simulink library "PC_Simulator_Lib"  (Simulink 8.2)
settings: Solver=ode45  StartTime=0.0  StopTime=10.0  RelTol=1e-3
values from neighbouring files (symbols this model uses):
  data = [r1 r2 r3 r4 L1 L2 L3 L4]    [strasse_Bedatung_HNI_ITI.m]
  distSameLane = 60    [InitialisationsEnv.m]
  eng_speed = [0 60 120 180 240 300 360 420 480 540 600 660 ... (101 elements, 1x101)]    [engine_table.mat]    (also in motor_parameter_calc.m = omega)
  Heading_init = 0    [Start.m]
  inertiaLateral = 25*(radiusWheel)^2    (= 4.129024)    [Start.m]
  laneWidth = 3.6    [InitialisationsEnv.m]    (also in strasse_Bedatung_HNI_ITI.m)
  omega_engine = [0.000000 150.000000 500.000000 1000.000000 1500.000000 2000.000000 2500.000000 3000.000000 3500.000000 4000.000000 4500.000000 5000.000000 5500.000000 6000.000000]    [friction_tables.m]
  omega_max = 6000    [engine_table.mat]    (also in motor_parameter_calc.m)
  omega_wheel = [0 20 40 60 80 100 122 143.7 164]    [friction_tables.m]
  para_Fellow_8_Points = ADAS.Fellow_8_Points    [ADAS_parameters.m]
  position_start_x = [x1 x2 x3 x4 x5 x6 x7]    [strasse_Bedatung_HNI_ITI.m]
  position_start_y = [y1 y2 y3 y4 y5 y6 y7]    [strasse_Bedatung_HNI_ITI.m]
  rad3rdLine = 57.2    [InitialisationsEnv.m]    (also in strasse_Bedatung_HNI_ITI.m)
  radiusWheel = 16*2.54/100    (= 0.4064)    [Start.m]
  s_values = [S1 S2 S3 S4 S5 S6 S7]    [strasse_Bedatung_HNI_ITI.m]
  segmentLimits = [segment1EndThirdLine                   segment2EndThirdLine                   segment3EndThirdLine                   segment4EndThirdLine                   segment5EndThirdLine                   segment6EndThirdLine                   segment7EndThirdLine                   segment8EndThirdLine                   ]    [InitialisationsEnv.m]    (also in strasse_Bedatung_HNI_ITI.m)
  setPosT = [-1.8 -5.4 -1.8 -5.4 -1.8 -5.4 -1.8 -5.4 -1.8 -5.4]    [InitialisationsEnv.m]
  torque = [297.089227105 300.997600937 304.800343044 308.497453426 312.088932082 315.574779014 318.95499422 322.229577701 325.398529457 328.461849487 331.419537793 334.271594373 ... (101 elements, 1x101)]    [engine_table.mat]    (also in motor_parameter_calc.m = g)
  Torque_lost = [0.000000 -8.777780 -15.000000 -26.800000 -29.600000 -32.700000 -35.900000 -39.300000 -42.800000 -46.500000 -50.300000 -54.300000 -58.500000 -62.800000 ]*0.6    [friction_tables.m]
  Torque_lost_wheel = [0.8 0.8 0.75 0.7 0.4 0.3 0.2 0.07 0.07]*0.2    [friction_tables.m]
  X_init = 0    [Start.m]
  Y_init = 1.8    [Start.m]
  Z_init = 0    [Start.m]
undefined symbols (not defined in the file or in its folder): Acc_Pedal, ADAS, Brake_Pedal, Joystick, Newton, Para, Raphson, Standard_Devices, Steering_Wheel_Angle, UDP_Protocol
libraries: simulink x43, rtwinlib x7, dspnetwork x2, simulink_extras x1, vrlib x1
(part 6 of 13)

== system PC_Simulator_Lib/Comunication_with_visualisation_Realtime/Subsystem2/Subsystem17 ==
  v[m|s] : Inport
  Gain : Gain  Gain=1/radiusWheel
  Integrator : Integrator
  Wheels_Rotation_Angle[rad] : Outport
  wires:
  Integrator/1 -> Wheels_Rotation_Angle[rad]/1
  v[m|s]/1 -> Gain/1
  Gain/1 -> Integrator/1

== system PC_Simulator_Lib/Comunication_with_visualisation_Realtime/Subsystem2/Subsystem18 ==
  v[m|s] : Inport
  Gain : Gain  Gain=1/radiusWheel
  Integrator : Integrator
  Wheels_Rotation_Angle[rad] : Outport
  wires:
  Gain/1 -> Integrator/1
  v[m|s]/1 -> Gain/1
  Integrator/1 -> Wheels_Rotation_Angle[rad]/1

== system PC_Simulator_Lib/Comunication_with_visualisation_Realtime/Subsystem2/Subsystem19 ==
  v[m|s] : Inport
  Gain : Gain  Gain=1/radiusWheel
  Integrator : Integrator
  Wheels_Rotation_Angle[rad] : Outport
  wires:
  Integrator/1 -> Wheels_Rotation_Angle[rad]/1
  v[m|s]/1 -> Gain/1
  Gain/1 -> Integrator/1

== system PC_Simulator_Lib/Comunication_with_visualisation_Realtime/Subsystem2/Subsystem2 ==
  In1 : Inport
  Constant9 : Constant  Value=Z_init
  Sum : Sum  Inputs=|++
  Out1 : Outport
  wires:
  In1/1 -> Sum/1
  Constant9/1 -> Sum/2
  Sum/1 -> Out1/1

== system PC_Simulator_Lib/Comunication_with_visualisation_Realtime/Subsystem2/Subsystem20 ==
  v[m|s] : Inport
  Gain : Gain  Gain=1/radiusWheel
  Integrator : Integrator
  Wheels_Rotation_Angle[rad] : Outport
  wires:
  Gain/1 -> Integrator/1
  v[m|s]/1 -> Gain/1
  Integrator/1 -> Wheels_Rotation_Angle[rad]/1

== system PC_Simulator_Lib/Comunication_with_visualisation_Realtime/Subsystem2/Subsystem3 ==
  FeedBack : Inport
  Mux : Mux  Inputs=14
  Terminator : Terminator
  zeros{7..10} (4 alike) : Constant  Value=0
  zeros12 : Constant
  Enablble_Fellow_Vehicles[bool] : Outport
  wires:
  Mux/1 -> Enablble_Fellow_Vehicles[bool]/1
  zeros12/1 -> Mux/2, Mux/6, Mux/7, Mux/8, Mux/9, Mux/10, Mux/5, Mux/4, Mux/3, Mux/1
  zeros7/1 -> Mux/12
  zeros8/1 -> Mux/11
  zeros9/1 -> Mux/14
  zeros10/1 -> Mux/13
  FeedBack/1 -> Terminator/1

== system PC_Simulator_Lib/Comunication_with_visualisation_Realtime/Subsystem2/Subsystem4 ==
  In1 : Inport
  Constant9 : Constant  Value=Z_init
  Sum : Sum  Inputs=|++
  Out1 : Outport
  wires:
  Sum/1 -> Out1/1
  Constant9/1 -> Sum/2
  In1/1 -> Sum/1

== system PC_Simulator_Lib/Comunication_with_visualisation_Realtime/Subsystem2/Subsystem5 ==
  In1 : Inport
  Constant9 : Constant  Value=Z_init
  Sum : Sum  Inputs=|++
  Out1 : Outport
  wires:
  In1/1 -> Sum/1
  Constant9/1 -> Sum/2
  Sum/1 -> Out1/1

== system PC_Simulator_Lib/Comunication_with_visualisation_Realtime/Subsystem2/Subsystem6 ==
  In1 : Inport
  Constant9 : Constant  Value=Z_init
  Sum : Sum  Inputs=|++
  Out1 : Outport
  wires:
  Sum/1 -> Out1/1
  Constant9/1 -> Sum/2
  In1/1 -> Sum/1

== system PC_Simulator_Lib/Comunication_with_visualisation_Realtime/Subsystem2/Subsystem7 ==
  In1 : Inport
  Constant9 : Constant  Value=Z_init
  Sum : Sum  Inputs=|++
  Out1 : Outport
  wires:
  In1/1 -> Sum/1
  Constant9/1 -> Sum/2
  Sum/1 -> Out1/1

== system PC_Simulator_Lib/Comunication_with_visualisation_Realtime/Subsystem2/Subsystem8 ==
  In1 : Inport
  Constant9 : Constant  Value=Z_init
  Sum : Sum  Inputs=|++
  Out1 : Outport
  wires:
  Sum/1 -> Out1/1
  Constant9/1 -> Sum/2
  In1/1 -> Sum/1

== system PC_Simulator_Lib/Comunication_with_visualisation_Realtime/Subsystem2/Subsystem9 ==
  In1 : Inport
  Constant9 : Constant  Value=Z_init
  Sum : Sum  Inputs=|++
  Out1 : Outport
  wires:
  In1/1 -> Sum/1
  Constant9/1 -> Sum/2
  Sum/1 -> Out1/1

== system PC_Simulator_Lib/Comunication_with_visualisation_Realtime_new_version/Maping_Block/Subsystem ==
  Vehicle_1_Vector : Inport
  Vehicle_2_Vector : Inport  Port=2
  Vehicle_3_Vector : Inport  Port=3
  Vehicle_4_Vector : Inport  Port=4
  Vehicle_5_Vector : Inport  Port=5
  Vehicle_6_Vector : Inport  Port=6
  Vehicle_7_Vector : Inport  Port=7
  Vehicle_8_Vector : Inport  Port=8
  Vehicle_9_Vector : Inport  Port=9
  Vehicle_10_Vector : Inport  Port=10
  Vehicle_11_Vector : Inport  Port=11
  Vehicle_12_Vector : Inport  Port=12
  Vehicle_13_Vector : Inport  Port=13
  Vehicle_14_Vector : Inport  Port=14
  Bus Creator : BusCreator  Inputs=14
  Bus Selector : BusSelector  OutputSignals=Vehicle_1_Vector.Vehicle_1_x[m],Vehicle_2_Vector.Vehicle_2_x[m],Vehicle_3_Vector.Vehicle_3_x[m],Vehicle_4_Vector3.Vehicle_4_x[m],Vehicle_5_Vector.Vehicle_5_x[m],Vehicle_6_Vector.Vehicle_6_x[m],Vehicle_7_Vector.Vehicle_7_x[m],Vehicle_8_Vector.Vehicle_8_x[m],Vehicle_9_Vector.Vehicle_9_x[m],Vehicle_10_Vector.Vehicle_10_x[m],Vehicle_11_Vector.Vehicle_11_x[m],Vehicle_12_Vector.Vehicle_12_x[m],Vehicle_13_Vector.Vehicle_13_x[m],Vehicle_14_Vector.Vehicle_14_x[m]
  Bus Selector1 : BusSelector  OutputSignals=Vehicle_1_Vector.Vehicle_1_y[m],Vehicle_2_Vector.Vehicle_2_y[m],Vehicle_3_Vector.Vehicle_3_y[m],Vehicle_4_Vector3.Vehicle_4_y[m],Vehicle_5_Vector.Vehicle_5_y[m],Vehicle_6_Vector.Vehicle_6_y[m],Vehicle_7_Vector.Vehicle_7_y[m],Vehicle_8_Vector.Vehicle_8_y[m],Vehicle_9_Vector.Vehicle_9_y[m],Vehicle_10_Vector.Vehicle_10_y[m],Vehicle_11_Vector.Vehicle_11_y[m],Vehicle_12_Vector.Vehicle_12_y[m],Vehicle_13_Vector.Vehicle_13_y[m],Vehicle_14_Vector.Vehicle_14_y[m]
  Bus Selector2 : BusSelector  OutputSignals=Vehicle_1_Vector.Vehicle_1_z[m],Vehicle_2_Vector.Vehicle_2_z[m],Vehicle_3_Vector.Vehicle_3_z[m],Vehicle_4_Vector3.Vehicle_4_z[m],Vehicle_5_Vector.Vehicle_5_z[m],Vehicle_6_Vector.Vehicle_6_z[m],Vehicle_7_Vector.Vehicle_7_z[m],Vehicle_8_Vector.Vehicle_8_z[m],Vehicle_9_Vector.Vehicle_9_z[m],Vehicle_10_Vector.Vehicle_10_z[m],Vehicle_11_Vector.Vehicle_11_z[m],Vehicle_12_Vector.Vehicle_12_z[m],Vehicle_13_Vector.Vehicle_13_z[m],Vehicle_14_Vector.Vehicle_14_z[m]
  Bus Selector3 : BusSelector  OutputSignals=Vehicle_1_Vector.Vehicle_1_Gear_Angle[deg],Vehicle_2_Vector.Vehicle_2_Gear_Angle[deg],Vehicle_3_Vector.Vehicle_3_Gear_Angle[deg],Vehicle_4_Vector3.Vehicle_4_Gear_Angle[deg],Vehicle_5_Vector.Vehicle_5_Gear_Angle[deg],Vehicle_6_Vector.Vehicle_6_Gear_Angle[deg],Vehicle_7_Vector.Vehicle_7_Gear_Angle[deg],Vehicle_8_Vector.Vehicle_8_Gear_Angle[deg],Vehicle_9_Vector.Vehicle_9_Gear_Angle[deg],Vehicle_10_Vector.Vehicle_10_Gear_Angle[deg],Vehicle_11_Vector.Vehicle_11_Gear_Angle[deg],Vehicle_12_Vector.Vehicle_12_Gear_Angle[deg],Vehicle_13_Vector.Vehicle_13_Gear_Angle[deg],Vehicle_14_Vector.Vehicle_14_Gear_Angle[deg]
  Bus Selector4 : BusSelector  OutputSignals=Vehicle_1_Vector.Vehicle_1_Wheels_Rotation_Angle[deg],Vehicle_2_Vector.Vehicle_2_Wheels_Rotation_Angle[deg],Vehicle_3_Vector.Vehicle_3_Wheels_Rotation_Angle[deg],Vehicle_4_Vector3.Vehicle_4_Wheels_Rotation_Angle[deg],Vehicle_5_Vector.Vehicle_5_Wheels_Rotation_Angle[deg],Vehicle_6_Vector.Vehicle_6_Wheels_Rotation_Angle[deg],Vehicle_7_Vector.Vehicle_7_Wheels_Rotation_Angle[deg],Vehicle_8_Vector.Vehicle_8_Wheels_Rotation_Angle[deg],Vehicle_9_Vector.Vehicle_9_Wheels_Rotation_Angle[deg],Vehicle_10_Vector.Vehicle_10_Wheels_Rotation_Angle[deg],Vehicle_11_Vector.Vehicle_11_Wheels_Rotation_Angle[deg],Vehicle_12_Vector.Vehicle_12_Wheels_Rotation_Angle[deg],Vehicle_13_Vector.Vehicle_13_Wheels_Rotation_Angle[deg],Vehicle_14_Vector.Vehicle_14_Wheels_Rotation_Angle[deg]
  Mux{,1..4} (5 alike) : Mux  Inputs=14
  Fellow_Vehicles_x_Vector_14[m] : Outport
  Fellow_Vehicles_y_Vector_14[m] : Outport  Port=2
  Fellow_Vehicles_z_Vector_14[m] : Outport  Port=3
  Fellow_Vehicles_Gear_Angle_Vector_14[deg] : Outport  Port=4
  Fellow_Vehicles_Wheel_Angle_Vector_14[deg] : Outport  Port=5
  wires:
  Mux4/1 -> Fellow_Vehicles_Wheel_Angle_Vector_14[deg]/1
  Mux3/1 -> Fellow_Vehicles_Gear_Angle_Vector_14[deg]/1
  Mux2/1 -> Fellow_Vehicles_z_Vector_14[m]/1
  Mux1/1 -> Fellow_Vehicles_y_Vector_14[m]/1
  Mux/1 -> Fellow_Vehicles_x_Vector_14[m]/1
  Bus Selector4/1 -> Mux4/1  "<Vehicle_1_Wheels_Rotation_Angle[deg]>"
  Bus Selector4/2 -> Mux4/2  "<Vehicle_2_Wheels_Rotation_Angle[deg]>"
  Bus Selector4/14 -> Mux4/14  "<Vehicle_14_Wheels_Rotation_Angle[deg]>"
  Bus Selector4/3 -> Mux4/3  "<Vehicle_3_Wheels_Rotation_Angle[deg]>"
  Bus Selector4/13 -> Mux4/13  "<Vehicle_13_Wheels_Rotation_Angle[deg]>"
  Bus Selector4/4 -> Mux4/4  "<Vehicle_4_Wheels_Rotation_Angle[deg]>"
  Bus Selector4/12 -> Mux4/12  "<Vehicle_12_Wheels_Rotation_Angle[deg]>"
  Bus Selector4/5 -> Mux4/5  "<Vehicle_5_Wheels_Rotation_Angle[deg]>"
  Bus Selector4/11 -> Mux4/11  "<Vehicle_11_Wheels_Rotation_Angle[deg]>"
  Bus Selector4/6 -> Mux4/6  "<Vehicle_6_Wheels_Rotation_Angle[deg]>"
  Bus Selector4/10 -> Mux4/10  "<Vehicle_10_Wheels_Rotation_Angle[deg]>"
  Bus Selector4/7 -> Mux4/7  "<Vehicle_7_Wheels_Rotation_Angle[deg]>"
  Bus Selector4/9 -> Mux4/9  "<Vehicle_9_Wheels_Rotation_Angle[deg]>"
  Bus Selector4/8 -> Mux4/8  "<Vehicle_8_Wheels_Rotation_Angle[deg]>"
  Bus Creator/1 -> Bus Selector/1, Bus Selector1/1, Bus Selector2/1, Bus Selector3/1, Bus Selector4/1
  Bus Selector3/1 -> Mux3/1  "<Vehicle_1_Gear_Angle[deg]>"
  Bus Selector3/2 -> Mux3/2  "<Vehicle_2_Gear_Angle[deg]>"
  Bus Selector3/14 -> Mux3/14  "<Vehicle_14_Gear_Angle[deg]>"
  Bus Selector3/3 -> Mux3/3  "<Vehicle_3_Gear_Angle[deg]>"
  Bus Selector3/13 -> Mux3/13  "<Vehicle_13_Gear_Angle[deg]>"
  Bus Selector3/4 -> Mux3/4  "<Vehicle_4_Gear_Angle[deg]>"
  Bus Selector3/12 -> Mux3/12  "<Vehicle_12_Gear_Angle[deg]>"
  Bus Selector3/5 -> Mux3/5  "<Vehicle_5_Gear_Angle[deg]>"
  Bus Selector3/11 -> Mux3/11  "<Vehicle_11_Gear_Angle[deg]>"
  Bus Selector3/6 -> Mux3/6  "<Vehicle_6_Gear_Angle[deg]>"
  Bus Selector3/10 -> Mux3/10  "<Vehicle_10_Gear_Angle[deg]>"
  Bus Selector3/7 -> Mux3/7  "<Vehicle_7_Gear_Angle[deg]>"
  Bus Selector3/9 -> Mux3/9  "<Vehicle_9_Gear_Angle[deg]>"
  Bus Selector3/8 -> Mux3/8  "<Vehicle_8_Gear_Angle[deg]>"
  Bus Selector2/1 -> Mux2/1  "<Vehicle_1_z[m]>"
  Bus Selector2/2 -> Mux2/2  "<Vehicle_2_z[m]>"
  Bus Selector2/14 -> Mux2/14  "<Vehicle_14_z[m]>"
  Bus Selector2/3 -> Mux2/3  "<Vehicle_3_z[m]>"
  Bus Selector2/13 -> Mux2/13  "<Vehicle_13_z[m]>"
  Bus Selector2/4 -> Mux2/4  "<Vehicle_4_z[m]>"
  Bus Selector2/12 -> Mux2/12  "<Vehicle_12_z[m]>"
  Bus Selector2/5 -> Mux2/5  "<Vehicle_5_z[m]>"
  Bus Selector2/11 -> Mux2/11  "<Vehicle_11_z[m]>"
  Bus Selector2/6 -> Mux2/6  "<Vehicle_6_z[m]>"
  Bus Selector2/10 -> Mux2/10  "<Vehicle_10_z[m]>"
  Bus Selector2/7 -> Mux2/7  "<Vehicle_7_z[m]>"
  Bus Selector2/9 -> Mux2/9  "<Vehicle_9_z[m]>"
  Bus Selector2/8 -> Mux2/8  "<Vehicle_8_z[m]>"
  Bus Selector1/1 -> Mux1/1  "<Vehicle_1_y[m]>"
  Bus Selector1/2 -> Mux1/2  "<Vehicle_2_y[m]>"
  Bus Selector1/14 -> Mux1/14  "<Vehicle_14_y[m]>"
  Bus Selector1/3 -> Mux1/3  "<Vehicle_3_y[m]>"
  Bus Selector1/13 -> Mux1/13  "<Vehicle_13_y[m]>"
  Bus Selector1/4 -> Mux1/4  "<Vehicle_4_y[m]>"
  Bus Selector1/12 -> Mux1/12  "<Vehicle_12_y[m]>"
  Bus Selector1/5 -> Mux1/5  "<Vehicle_5_y[m]>"
  Bus Selector1/11 -> Mux1/11  "<Vehicle_11_y[m]>"
  Bus Selector1/6 -> Mux1/6  "<Vehicle_6_y[m]>"
  Bus Selector1/10 -> Mux1/10  "<Vehicle_10_y[m]>"
  Bus Selector1/7 -> Mux1/7  "<Vehicle_7_y[m]>"
  Bus Selector1/9 -> Mux1/9  "<Vehicle_9_y[m]>"
  Bus Selector1/8 -> Mux1/8  "<Vehicle_8_y[m]>"
  Bus Selector/1 -> Mux/1  "<Vehicle_1_x[m]>"
  Bus Selector/2 -> Mux/2  "<Vehicle_2_x[m]>"
  Bus Selector/14 -> Mux/14  "<Vehicle_14_x[m]>"
  Bus Selector/3 -> Mux/3  "<Vehicle_3_x[m]>"
  Bus Selector/13 -> Mux/13  "<Vehicle_13_x[m]>"
  Bus Selector/4 -> Mux/4  "<Vehicle_4_x[m]>"
  Bus Selector/12 -> Mux/12  "<Vehicle_12_x[m]>"
  Bus Selector/5 -> Mux/5  "<Vehicle_5_x[m]>"
  Bus Selector/11 -> Mux/11  "<Vehicle_11_x[m]>"
  Bus Selector/6 -> Mux/6  "<Vehicle_6_x[m]>"
  Bus Selector/10 -> Mux/10  "<Vehicle_10_x[m]>"
  Bus Selector/7 -> Mux/7  "<Vehicle_7_x[m]>"
  Bus Selector/9 -> Mux/9  "<Vehicle_9_x[m]>"
  Bus Selector/8 -> Mux/8  "<Vehicle_8_x[m]>"
  Vehicle_14_Vector/1 -> Bus Creator/14
  Vehicle_12_Vector/1 -> Bus Creator/12
  Vehicle_11_Vector/1 -> Bus Creator/11
  Vehicle_9_Vector/1 -> Bus Creator/9
  Vehicle_10_Vector/1 -> Bus Creator/10
  Vehicle_13_Vector/1 -> Bus Creator/13
  Vehicle_8_Vector/1 -> Bus Creator/8
  Vehicle_7_Vector/1 -> Bus Creator/7
  Vehicle_6_Vector/1 -> Bus Creator/6
  Vehicle_5_Vector/1 -> Bus Creator/5
  Vehicle_4_Vector/1 -> Bus Creator/4
  Vehicle_3_Vector/1 -> Bus Creator/3
  Vehicle_2_Vector/1 -> Bus Creator/2
  Vehicle_1_Vector/1 -> Bus Creator/1

== system PC_Simulator_Lib/Comunication_with_visualisation_Realtime_new_version/Subsystem2/Subsystem ==
  In1 : Inport
  Constant9 : Constant  Value=0.8
  Sum : Sum  Inputs=|++
  Out1 : Outport
  wires:
  Sum/1 -> Out1/1
  Constant9/1 -> Sum/2
  In1/1 -> Sum/1

== system PC_Simulator_Lib/Comunication_with_visualisation_Realtime_new_version/Subsystem2/Subsystem1 ==
  In1 : Inport
  Constant9 : Constant  Value=Z_init
  Sum : Sum  Inputs=|++
  Out1 : Outport
  wires:
  In1/1 -> Sum/1
  Constant9/1 -> Sum/2
  Sum/1 -> Out1/1

== system PC_Simulator_Lib/Comunication_with_visualisation_Realtime_new_version/Subsystem2/Subsystem10 ==
  In1 : Inport
  Constant9 : Constant  Value=Z_init
  Sum : Sum  Inputs=|++
  Out1 : Outport
  wires:
  In1/1 -> Sum/1
  Constant9/1 -> Sum/2
  Sum/1 -> Out1/1

== system PC_Simulator_Lib/Comunication_with_visualisation_Realtime_new_version/Subsystem2/Subsystem11 ==
  v[m|s] : Inport
  Gain : Gain  Gain=1/radiusWheel
  Integrator : Integrator
  Wheels_Rotation_Angle[rad] : Outport
  wires:
  Gain/1 -> Integrator/1
  v[m|s]/1 -> Gain/1
  Integrator/1 -> Wheels_Rotation_Angle[rad]/1

== system PC_Simulator_Lib/Comunication_with_visualisation_Realtime_new_version/Subsystem2/Subsystem12 ==
  v[m|s] : Inport
  Gain : Gain  Gain=1/radiusWheel
  Integrator : Integrator
  Wheels_Rotation_Angle[rad] : Outport
  wires:
  Integrator/1 -> Wheels_Rotation_Angle[rad]/1
  v[m|s]/1 -> Gain/1
  Gain/1 -> Integrator/1

== system PC_Simulator_Lib/Comunication_with_visualisation_Realtime_new_version/Subsystem2/Subsystem13 ==
  v[m|s] : Inport
  Gain : Gain  Gain=1/radiusWheel
  Integrator : Integrator
  Wheels_Rotation_Angle[rad] : Outport
  wires:
  Gain/1 -> Integrator/1
  v[m|s]/1 -> Gain/1
  Integrator/1 -> Wheels_Rotation_Angle[rad]/1

== system PC_Simulator_Lib/Comunication_with_visualisation_Realtime_new_version/Subsystem2/Subsystem14 ==
  v[m|s] : Inport
  Gain : Gain  Gain=1/radiusWheel
  Integrator : Integrator
  Wheels_Rotation_Angle[rad] : Outport
  wires:
  Integrator/1 -> Wheels_Rotation_Angle[rad]/1
  v[m|s]/1 -> Gain/1
  Gain/1 -> Integrator/1

== system PC_Simulator_Lib/Comunication_with_visualisation_Realtime_new_version/Subsystem2/Subsystem15 ==
  v[m|s] : Inport
  Gain : Gain  Gain=1/radiusWheel
  Integrator : Integrator
  Wheels_Rotation_Angle[rad] : Outport
  wires:
  Gain/1 -> Integrator/1
  v[m|s]/1 -> Gain/1
  Integrator/1 -> Wheels_Rotation_Angle[rad]/1

== system PC_Simulator_Lib/Comunication_with_visualisation_Realtime_new_version/Subsystem2/Subsystem16 ==
  v[m|s] : Inport
  Gain : Gain  Gain=1/radiusWheel
  Integrator : Integrator
  Wheels_Rotation_Angle[rad] : Outport
  wires:
  Integrator/1 -> Wheels_Rotation_Angle[rad]/1
  v[m|s]/1 -> Gain/1
  Gain/1 -> Integrator/1

== system PC_Simulator_Lib/Comunication_with_visualisation_Realtime_new_version/Subsystem2/Subsystem17 ==
  v[m|s] : Inport
  Gain : Gain  Gain=1/radiusWheel
  Integrator : Integrator
  Wheels_Rotation_Angle[rad] : Outport
  wires:
  Gain/1 -> Integrator/1
  v[m|s]/1 -> Gain/1
  Integrator/1 -> Wheels_Rotation_Angle[rad]/1

== system PC_Simulator_Lib/Comunication_with_visualisation_Realtime_new_version/Subsystem2/Subsystem18 ==
  v[m|s] : Inport
  Gain : Gain  Gain=1/radiusWheel
  Integrator : Integrator
  Wheels_Rotation_Angle[rad] : Outport
  wires:
  Integrator/1 -> Wheels_Rotation_Angle[rad]/1
  v[m|s]/1 -> Gain/1
  Gain/1 -> Integrator/1

== system PC_Simulator_Lib/Comunication_with_visualisation_Realtime_new_version/Subsystem2/Subsystem19 ==
  v[m|s] : Inport
  Gain : Gain  Gain=1/radiusWheel
  Integrator : Integrator
  Wheels_Rotation_Angle[rad] : Outport
  wires:
  Gain/1 -> Integrator/1
  v[m|s]/1 -> Gain/1
  Integrator/1 -> Wheels_Rotation_Angle[rad]/1

== system PC_Simulator_Lib/Comunication_with_visualisation_Realtime_new_version/Subsystem2/Subsystem2 ==
  In1 : Inport
  Constant9 : Constant  Value=Z_init
  Sum : Sum  Inputs=|++
  Out1 : Outport
  wires:
  Sum/1 -> Out1/1
  Constant9/1 -> Sum/2
  In1/1 -> Sum/1

== system PC_Simulator_Lib/Comunication_with_visualisation_Realtime_new_version/Subsystem2/Subsystem20 ==
  v[m|s] : Inport
  Gain : Gain  Gain=1/radiusWheel
  Integrator : Integrator
  Wheels_Rotation_Angle[rad] : Outport
  wires:
  Integrator/1 -> Wheels_Rotation_Angle[rad]/1
  v[m|s]/1 -> Gain/1
  Gain/1 -> Integrator/1

== system PC_Simulator_Lib/Comunication_with_visualisation_Realtime_new_version/Subsystem2/Subsystem4 ==
  In1 : Inport
  Constant9 : Constant  Value=Z_init
  Sum : Sum  Inputs=|++
  Out1 : Outport
  wires:
  In1/1 -> Sum/1
  Constant9/1 -> Sum/2
  Sum/1 -> Out1/1

== system PC_Simulator_Lib/Comunication_with_visualisation_Realtime_new_version/Subsystem2/Subsystem5 ==
  In1 : Inport
  Constant9 : Constant  Value=Z_init
  Sum : Sum  Inputs=|++
  Out1 : Outport
  wires:
  Sum/1 -> Out1/1
  Constant9/1 -> Sum/2
  In1/1 -> Sum/1

== system PC_Simulator_Lib/Comunication_with_visualisation_Realtime_new_version/Subsystem2/Subsystem6 ==
  In1 : Inport
  Constant9 : Constant  Value=Z_init
  Sum : Sum  Inputs=|++
  Out1 : Outport
  wires:
  In1/1 -> Sum/1
  Constant9/1 -> Sum/2
  Sum/1 -> Out1/1

== system PC_Simulator_Lib/Comunication_with_visualisation_Realtime_new_version/Subsystem2/Subsystem7 ==
  In1 : Inport
  Constant9 : Constant  Value=Z_init
  Sum : Sum  Inputs=|++
  Out1 : Outport
  wires:
  Sum/1 -> Out1/1
  Constant9/1 -> Sum/2
  In1/1 -> Sum/1

== system PC_Simulator_Lib/Comunication_with_visualisation_Realtime_new_version/Subsystem2/Subsystem8 ==
  In1 : Inport
  Constant9 : Constant  Value=Z_init
  Sum : Sum  Inputs=|++
  Out1 : Outport
  wires:
  In1/1 -> Sum/1
  Constant9/1 -> Sum/2
  Sum/1 -> Out1/1

== system PC_Simulator_Lib/Comunication_with_visualisation_Realtime_new_version/Subsystem2/Subsystem9 ==
  In1 : Inport
  Constant9 : Constant  Value=Z_init
  Sum : Sum  Inputs=|++
  Out1 : Outport
  wires:
  Sum/1 -> Out1/1
  Constant9/1 -> Sum/2
  In1/1 -> Sum/1

== system PC_Simulator_Lib/Comunication_with_visualisation_normal_mode/Maping_Block/Subsystem ==
  Vehicle_1_Vector : Inport
  Vehicle_2_Vector : Inport  Port=2
  Vehicle_3_Vector : Inport  Port=3
  Vehicle_4_Vector : Inport  Port=4
  Vehicle_5_Vector : Inport  Port=5
  Vehicle_6_Vector : Inport  Port=6
  Vehicle_7_Vector : Inport  Port=7
  Vehicle_8_Vector : Inport  Port=8
  Vehicle_9_Vector : Inport  Port=9
  Vehicle_10_Vector : Inport  Port=10
  Vehicle_11_Vector : Inport  Port=11
  Vehicle_12_Vector : Inport  Port=12
  Vehicle_13_Vector : Inport  Port=13
  Vehicle_14_Vector : Inport  Port=14
  Bus Creator : BusCreator  Inputs=14
  Bus Selector : BusSelector  OutputSignals=Vehicle_1_Vector.Vehicle_1_x[m],Vehicle_2_Vector.Vehicle_2_x[m],Vehicle_3_Vector.Vehicle_3_x[m],Vehicle_4_Vector3.Vehicle_4_x[m],Vehicle_5_Vector.Vehicle_5_x[m],Vehicle_6_Vector.Vehicle_6_x[m],Vehicle_7_Vector.Vehicle_7_x[m],Vehicle_8_Vector.Vehicle_8_x[m],Vehicle_9_Vector.Vehicle_9_x[m],Vehicle_10_Vector.Vehicle_10_x[m],Vehicle_11_Vector.Vehicle_11_x[m],Vehicle_12_Vector.Vehicle_12_x[m],Vehicle_13_Vector.Vehicle_13_x[m],Vehicle_14_Vector.Vehicle_14_x[m]
  Bus Selector1 : BusSelector  OutputSignals=Vehicle_1_Vector.Vehicle_1_y[m],Vehicle_2_Vector.Vehicle_2_y[m],Vehicle_3_Vector.Vehicle_3_y[m],Vehicle_4_Vector3.Vehicle_4_y[m],Vehicle_5_Vector.Vehicle_5_y[m],Vehicle_6_Vector.Vehicle_6_y[m],Vehicle_7_Vector.Vehicle_7_y[m],Vehicle_8_Vector.Vehicle_8_y[m],Vehicle_9_Vector.Vehicle_9_y[m],Vehicle_10_Vector.Vehicle_10_y[m],Vehicle_11_Vector.Vehicle_11_y[m],Vehicle_12_Vector.Vehicle_12_y[m],Vehicle_13_Vector.Vehicle_13_y[m],Vehicle_14_Vector.Vehicle_14_y[m]
  Bus Selector2 : BusSelector  OutputSignals=Vehicle_1_Vector.Vehicle_1_z[m],Vehicle_2_Vector.Vehicle_2_z[m],Vehicle_3_Vector.Vehicle_3_z[m],Vehicle_4_Vector3.Vehicle_4_z[m],Vehicle_5_Vector.Vehicle_5_z[m],Vehicle_6_Vector.Vehicle_6_z[m],Vehicle_7_Vector.Vehicle_7_z[m],Vehicle_8_Vector.Vehicle_8_z[m],Vehicle_9_Vector.Vehicle_9_z[m],Vehicle_10_Vector.Vehicle_10_z[m],Vehicle_11_Vector.Vehicle_11_z[m],Vehicle_12_Vector.Vehicle_12_z[m],Vehicle_13_Vector.Vehicle_13_z[m],Vehicle_14_Vector.Vehicle_14_z[m]
  Bus Selector3 : BusSelector  OutputSignals=Vehicle_1_Vector.Vehicle_1_Gear_Angle[deg],Vehicle_2_Vector.Vehicle_2_Gear_Angle[deg],Vehicle_3_Vector.Vehicle_3_Gear_Angle[deg],Vehicle_4_Vector3.Vehicle_4_Gear_Angle[deg],Vehicle_5_Vector.Vehicle_5_Gear_Angle[deg],Vehicle_6_Vector.Vehicle_6_Gear_Angle[deg],Vehicle_7_Vector.Vehicle_7_Gear_Angle[deg],Vehicle_8_Vector.Vehicle_8_Gear_Angle[deg],Vehicle_9_Vector.Vehicle_9_Gear_Angle[deg],Vehicle_10_Vector.Vehicle_10_Gear_Angle[deg],Vehicle_11_Vector.Vehicle_11_Gear_Angle[deg],Vehicle_12_Vector.Vehicle_12_Gear_Angle[deg],Vehicle_13_Vector.Vehicle_13_Gear_Angle[deg],Vehicle_14_Vector.Vehicle_14_Gear_Angle[deg]
  Bus Selector4 : BusSelector  OutputSignals=Vehicle_1_Vector.Vehicle_1_Wheels_Rotation_Angle[deg],Vehicle_2_Vector.Vehicle_2_Wheels_Rotation_Angle[deg],Vehicle_3_Vector.Vehicle_3_Wheels_Rotation_Angle[deg],Vehicle_4_Vector3.Vehicle_4_Wheels_Rotation_Angle[deg],Vehicle_5_Vector.Vehicle_5_Wheels_Rotation_Angle[deg],Vehicle_6_Vector.Vehicle_6_Wheels_Rotation_Angle[deg],Vehicle_7_Vector.Vehicle_7_Wheels_Rotation_Angle[deg],Vehicle_8_Vector.Vehicle_8_Wheels_Rotation_Angle[deg],Vehicle_9_Vector.Vehicle_9_Wheels_Rotation_Angle[deg],Vehicle_10_Vector.Vehicle_10_Wheels_Rotation_Angle[deg],Vehicle_11_Vector.Vehicle_11_Wheels_Rotation_Angle[deg],Vehicle_12_Vector.Vehicle_12_Wheels_Rotation_Angle[deg],Vehicle_13_Vector.Vehicle_13_Wheels_Rotation_Angle[deg],Vehicle_14_Vector.Vehicle_14_Wheels_Rotation_Angle[deg]
  Mux{,1..4} (5 alike) : Mux  Inputs=14
  Fellow_Vehicles_x_Vector_14[m] : Outport
  Fellow_Vehicles_y_Vector_14[m] : Outport  Port=2
  Fellow_Vehicles_z_Vector_14[m] : Outport  Port=3
  Fellow_Vehicles_Gear_Angle_Vector_14[deg] : Outport  Port=4
  Fellow_Vehicles_Wheel_Angle_Vector_14[deg] : Outport  Port=5
  wires:
  Vehicle_1_Vector/1 -> Bus Creator/1
  Vehicle_2_Vector/1 -> Bus Creator/2
  Vehicle_3_Vector/1 -> Bus Creator/3
  Vehicle_4_Vector/1 -> Bus Creator/4
  Vehicle_5_Vector/1 -> Bus Creator/5
  Vehicle_6_Vector/1 -> Bus Creator/6
  Vehicle_7_Vector/1 -> Bus Creator/7
  Vehicle_8_Vector/1 -> Bus Creator/8
  Vehicle_13_Vector/1 -> Bus Creator/13
  Vehicle_10_Vector/1 -> Bus Creator/10
  Vehicle_9_Vector/1 -> Bus Creator/9
  Vehicle_11_Vector/1 -> Bus Creator/11
  Vehicle_12_Vector/1 -> Bus Creator/12
  Vehicle_14_Vector/1 -> Bus Creator/14
  Bus Selector/8 -> Mux/8  "<Vehicle_8_x[m]>"
  Bus Selector/9 -> Mux/9  "<Vehicle_9_x[m]>"
  Bus Selector/7 -> Mux/7  "<Vehicle_7_x[m]>"
  Bus Selector/10 -> Mux/10  "<Vehicle_10_x[m]>"
  Bus Selector/6 -> Mux/6  "<Vehicle_6_x[m]>"
  Bus Selector/11 -> Mux/11  "<Vehicle_11_x[m]>"
  Bus Selector/5 -> Mux/5  "<Vehicle_5_x[m]>"
  Bus Selector/12 -> Mux/12  "<Vehicle_12_x[m]>"
  Bus Selector/4 -> Mux/4  "<Vehicle_4_x[m]>"
  Bus Selector/13 -> Mux/13  "<Vehicle_13_x[m]>"
  Bus Selector/3 -> Mux/3  "<Vehicle_3_x[m]>"
  Bus Selector/14 -> Mux/14  "<Vehicle_14_x[m]>"
  Bus Selector/2 -> Mux/2  "<Vehicle_2_x[m]>"
  Bus Selector/1 -> Mux/1  "<Vehicle_1_x[m]>"
  Bus Selector1/8 -> Mux1/8  "<Vehicle_8_y[m]>"
  Bus Selector1/9 -> Mux1/9  "<Vehicle_9_y[m]>"
  Bus Selector1/7 -> Mux1/7  "<Vehicle_7_y[m]>"
  Bus Selector1/10 -> Mux1/10  "<Vehicle_10_y[m]>"
  Bus Selector1/6 -> Mux1/6  "<Vehicle_6_y[m]>"
  Bus Selector1/11 -> Mux1/11  "<Vehicle_11_y[m]>"
  Bus Selector1/5 -> Mux1/5  "<Vehicle_5_y[m]>"
  Bus Selector1/12 -> Mux1/12  "<Vehicle_12_y[m]>"
  Bus Selector1/4 -> Mux1/4  "<Vehicle_4_y[m]>"
  Bus Selector1/13 -> Mux1/13  "<Vehicle_13_y[m]>"
  Bus Selector1/3 -> Mux1/3  "<Vehicle_3_y[m]>"
  Bus Selector1/14 -> Mux1/14  "<Vehicle_14_y[m]>"
  Bus Selector1/2 -> Mux1/2  "<Vehicle_2_y[m]>"
  Bus Selector1/1 -> Mux1/1  "<Vehicle_1_y[m]>"
  Bus Selector2/8 -> Mux2/8  "<Vehicle_8_z[m]>"
  Bus Selector2/9 -> Mux2/9  "<Vehicle_9_z[m]>"
  Bus Selector2/7 -> Mux2/7  "<Vehicle_7_z[m]>"
  Bus Selector2/10 -> Mux2/10  "<Vehicle_10_z[m]>"
  Bus Selector2/6 -> Mux2/6  "<Vehicle_6_z[m]>"
  Bus Selector2/11 -> Mux2/11  "<Vehicle_11_z[m]>"
  Bus Selector2/5 -> Mux2/5  "<Vehicle_5_z[m]>"
  Bus Selector2/12 -> Mux2/12  "<Vehicle_12_z[m]>"
  Bus Selector2/4 -> Mux2/4  "<Vehicle_4_z[m]>"
  Bus Selector2/13 -> Mux2/13  "<Vehicle_13_z[m]>"
  Bus Selector2/3 -> Mux2/3  "<Vehicle_3_z[m]>"
  Bus Selector2/14 -> Mux2/14  "<Vehicle_14_z[m]>"
  Bus Selector2/2 -> Mux2/2  "<Vehicle_2_z[m]>"
  Bus Selector2/1 -> Mux2/1  "<Vehicle_1_z[m]>"
  Bus Selector3/8 -> Mux3/8  "<Vehicle_8_Gear_Angle[deg]>"
  Bus Selector3/9 -> Mux3/9  "<Vehicle_9_Gear_Angle[deg]>"
  Bus Selector3/7 -> Mux3/7  "<Vehicle_7_Gear_Angle[deg]>"
  Bus Selector3/10 -> Mux3/10  "<Vehicle_10_Gear_Angle[deg]>"
  Bus Selector3/6 -> Mux3/6  "<Vehicle_6_Gear_Angle[deg]>"
  Bus Selector3/11 -> Mux3/11  "<Vehicle_11_Gear_Angle[deg]>"
  Bus Selector3/5 -> Mux3/5  "<Vehicle_5_Gear_Angle[deg]>"
  Bus Selector3/12 -> Mux3/12  "<Vehicle_12_Gear_Angle[deg]>"
  Bus Selector3/4 -> Mux3/4  "<Vehicle_4_Gear_Angle[deg]>"
  Bus Selector3/13 -> Mux3/13  "<Vehicle_13_Gear_Angle[deg]>"
  Bus Selector3/3 -> Mux3/3  "<Vehicle_3_Gear_Angle[deg]>"
  Bus Selector3/14 -> Mux3/14  "<Vehicle_14_Gear_Angle[deg]>"
  Bus Selector3/2 -> Mux3/2  "<Vehicle_2_Gear_Angle[deg]>"
  Bus Selector3/1 -> Mux3/1  "<Vehicle_1_Gear_Angle[deg]>"
  Bus Creator/1 -> Bus Selector4/1, Bus Selector3/1, Bus Selector2/1, Bus Selector1/1, Bus Selector/1
  Bus Selector4/8 -> Mux4/8  "<Vehicle_8_Wheels_Rotation_Angle[deg]>"
  Bus Selector4/9 -> Mux4/9  "<Vehicle_9_Wheels_Rotation_Angle[deg]>"
  Bus Selector4/7 -> Mux4/7  "<Vehicle_7_Wheels_Rotation_Angle[deg]>"
  Bus Selector4/10 -> Mux4/10  "<Vehicle_10_Wheels_Rotation_Angle[deg]>"
  Bus Selector4/6 -> Mux4/6  "<Vehicle_6_Wheels_Rotation_Angle[deg]>"
  Bus Selector4/11 -> Mux4/11  "<Vehicle_11_Wheels_Rotation_Angle[deg]>"
  Bus Selector4/5 -> Mux4/5  "<Vehicle_5_Wheels_Rotation_Angle[deg]>"
  Bus Selector4/12 -> Mux4/12  "<Vehicle_12_Wheels_Rotation_Angle[deg]>"
  Bus Selector4/4 -> Mux4/4  "<Vehicle_4_Wheels_Rotation_Angle[deg]>"
  Bus Selector4/13 -> Mux4/13  "<Vehicle_13_Wheels_Rotation_Angle[deg]>"
  Bus Selector4/3 -> Mux4/3  "<Vehicle_3_Wheels_Rotation_Angle[deg]>"
  Bus Selector4/14 -> Mux4/14  "<Vehicle_14_Wheels_Rotation_Angle[deg]>"
  Bus Selector4/2 -> Mux4/2  "<Vehicle_2_Wheels_Rotation_Angle[deg]>"
  Bus Selector4/1 -> Mux4/1  "<Vehicle_1_Wheels_Rotation_Angle[deg]>"
  Mux/1 -> Fellow_Vehicles_x_Vector_14[m]/1
  Mux1/1 -> Fellow_Vehicles_y_Vector_14[m]/1
  Mux2/1 -> Fellow_Vehicles_z_Vector_14[m]/1
  Mux3/1 -> Fellow_Vehicles_Gear_Angle_Vector_14[deg]/1
  Mux4/1 -> Fellow_Vehicles_Wheel_Angle_Vector_14[deg]/1

== system PC_Simulator_Lib/Comunication_with_visualisation_normal_mode/Subsystem2/Subsystem ==
  In1 : Inport
  Constant9 : Constant  Value=Z_init
  Sum : Sum  Inputs=|++
  Out1 : Outport
  wires:
  In1/1 -> Sum/1
  Constant9/1 -> Sum/2
  Sum/1 -> Out1/1

== system PC_Simulator_Lib/Comunication_with_visualisation_normal_mode/Subsystem2/Subsystem1 ==
  In1 : Inport
  Constant9 : Constant  Value=Z_init
  Sum : Sum  Inputs=|++
  Out1 : Outport
  wires:
  Sum/1 -> Out1/1
  Constant9/1 -> Sum/2
  In1/1 -> Sum/1

== system PC_Simulator_Lib/Comunication_with_visualisation_normal_mode/Subsystem2/Subsystem10 ==
  In1 : Inport
  Constant9 : Constant  Value=Z_init
  Sum : Sum  Inputs=|++
  Out1 : Outport
  wires:
  Sum/1 -> Out1/1
  Constant9/1 -> Sum/2
  In1/1 -> Sum/1

== system PC_Simulator_Lib/Comunication_with_visualisation_normal_mode/Subsystem2/Subsystem11 ==
  v[m|s] : Inport
  Gain : Gain  Gain=1/radiusWheel
  Integrator : Integrator
  Wheels_Rotation_Angle[rad] : Outport
  wires:
  Integrator/1 -> Wheels_Rotation_Angle[rad]/1
  v[m|s]/1 -> Gain/1
  Gain/1 -> Integrator/1

== system PC_Simulator_Lib/Comunication_with_visualisation_normal_mode/Subsystem2/Subsystem12 ==
  v[m|s] : Inport
  Gain : Gain  Gain=1/radiusWheel
  Integrator : Integrator
  Wheels_Rotation_Angle[rad] : Outport
  wires:
  Gain/1 -> Integrator/1
  v[m|s]/1 -> Gain/1
  Integrator/1 -> Wheels_Rotation_Angle[rad]/1

== system PC_Simulator_Lib/Comunication_with_visualisation_normal_mode/Subsystem2/Subsystem13 ==
  v[m|s] : Inport
  Gain : Gain  Gain=1/radiusWheel
  Integrator : Integrator
  Wheels_Rotation_Angle[rad] : Outport
  wires:
  Integrator/1 -> Wheels_Rotation_Angle[rad]/1
  v[m|s]/1 -> Gain/1
  Gain/1 -> Integrator/1

== system PC_Simulator_Lib/Comunication_with_visualisation_normal_mode/Subsystem2/Subsystem14 ==
  v[m|s] : Inport
  Gain : Gain  Gain=1/radiusWheel
  Integrator : Integrator
  Wheels_Rotation_Angle[rad] : Outport
  wires:
  Gain/1 -> Integrator/1
  v[m|s]/1 -> Gain/1
  Integrator/1 -> Wheels_Rotation_Angle[rad]/1

== system PC_Simulator_Lib/Comunication_with_visualisation_normal_mode/Subsystem2/Subsystem15 ==
  v[m|s] : Inport
  Gain : Gain  Gain=1/radiusWheel
  Integrator : Integrator
  Wheels_Rotation_Angle[rad] : Outport
  wires:
  Integrator/1 -> Wheels_Rotation_Angle[rad]/1
  v[m|s]/1 -> Gain/1
  Gain/1 -> Integrator/1

== system PC_Simulator_Lib/Comunication_with_visualisation_normal_mode/Subsystem2/Subsystem16 ==
  v[m|s] : Inport
  Gain : Gain  Gain=1/radiusWheel
  Integrator : Integrator
  Wheels_Rotation_Angle[rad] : Outport
  wires:
  Gain/1 -> Integrator/1
  v[m|s]/1 -> Gain/1
  Integrator/1 -> Wheels_Rotation_Angle[rad]/1

== system PC_Simulator_Lib/Comunication_with_visualisation_normal_mode/Subsystem2/Subsystem17 ==
  v[m|s] : Inport
  Gain : Gain  Gain=1/radiusWheel
  Integrator : Integrator
  Wheels_Rotation_Angle[rad] : Outport
  wires:
  Integrator/1 -> Wheels_Rotation_Angle[rad]/1
  v[m|s]/1 -> Gain/1
  Gain/1 -> Integrator/1

== system PC_Simulator_Lib/Comunication_with_visualisation_normal_mode/Subsystem2/Subsystem18 ==
  v[m|s] : Inport
  Gain : Gain  Gain=1/radiusWheel
  Integrator : Integrator
  Wheels_Rotation_Angle[rad] : Outport
  wires:
  Gain/1 -> Integrator/1
  v[m|s]/1 -> Gain/1
  Integrator/1 -> Wheels_Rotation_Angle[rad]/1

== system PC_Simulator_Lib/Comunication_with_visualisation_normal_mode/Subsystem2/Subsystem19 ==
  v[m|s] : Inport
  Gain : Gain  Gain=1/radiusWheel
  Integrator : Integrator
  Wheels_Rotation_Angle[rad] : Outport
  wires:
  Integrator/1 -> Wheels_Rotation_Angle[rad]/1
  v[m|s]/1 -> Gain/1
  Gain/1 -> Integrator/1

== system PC_Simulator_Lib/Comunication_with_visualisation_normal_mode/Subsystem2/Subsystem2 ==
  In1 : Inport
  Constant9 : Constant  Value=Z_init
  Sum : Sum  Inputs=|++
  Out1 : Outport
  wires:
  In1/1 -> Sum/1
  Constant9/1 -> Sum/2
  Sum/1 -> Out1/1

== system PC_Simulator_Lib/Comunication_with_visualisation_normal_mode/Subsystem2/Subsystem20 ==
  v[m|s] : Inport
  Gain : Gain  Gain=1/radiusWheel
  Integrator : Integrator
  Wheels_Rotation_Angle[rad] : Outport
  wires:
  Gain/1 -> Integrator/1
  v[m|s]/1 -> Gain/1
  Integrator/1 -> Wheels_Rotation_Angle[rad]/1

== system PC_Simulator_Lib/Comunication_with_visualisation_normal_mode/Subsystem2/Subsystem3 ==
  FeedBack : Inport
  Mux : Mux  Inputs=14
  Terminator : Terminator
  zeros{7..10} (4 alike) : Constant  Value=0
  zeros12 : Constant
  Enablble_Fellow_Vehicles[bool] : Outport
  wires:
  Mux/1 -> Enablble_Fellow_Vehicles[bool]/1
  zeros12/1 -> Mux/2, Mux/6, Mux/7, Mux/8, Mux/9, Mux/10, Mux/5, Mux/4, Mux/3, Mux/1
  zeros7/1 -> Mux/12
  zeros8/1 -> Mux/11
  zeros9/1 -> Mux/14
  zeros10/1 -> Mux/13
  FeedBack/1 -> Terminator/1

== system PC_Simulator_Lib/Comunication_with_visualisation_normal_mode/Subsystem2/Subsystem4 ==
  In1 : Inport
  Constant9 : Constant  Value=Z_init
  Sum : Sum  Inputs=|++
  Out1 : Outport
  wires:
  Sum/1 -> Out1/1
  Constant9/1 -> Sum/2
  In1/1 -> Sum/1

== system PC_Simulator_Lib/Comunication_with_visualisation_normal_mode/Subsystem2/Subsystem5 ==
  In1 : Inport
  Constant9 : Constant  Value=Z_init
  Sum : Sum  Inputs=|++
  Out1 : Outport
  wires:
  In1/1 -> Sum/1
  Constant9/1 -> Sum/2
  Sum/1 -> Out1/1

== system PC_Simulator_Lib/Comunication_with_visualisation_normal_mode/Subsystem2/Subsystem6 ==
  In1 : Inport
  Constant9 : Constant  Value=Z_init
  Sum : Sum  Inputs=|++
  Out1 : Outport
  wires:
  Sum/1 -> Out1/1
  Constant9/1 -> Sum/2
  In1/1 -> Sum/1

== system PC_Simulator_Lib/Comunication_with_visualisation_normal_mode/Subsystem2/Subsystem7 ==
  In1 : Inport
  Constant9 : Constant  Value=Z_init
  Sum : Sum  Inputs=|++
  Out1 : Outport
  wires:
  In1/1 -> Sum/1
  Constant9/1 -> Sum/2
  Sum/1 -> Out1/1

== system PC_Simulator_Lib/Comunication_with_visualisation_normal_mode/Subsystem2/Subsystem8 ==
  In1 : Inport
  Constant9 : Constant  Value=Z_init
  Sum : Sum  Inputs=|++
  Out1 : Outport
  wires:
  Sum/1 -> Out1/1
  Constant9/1 -> Sum/2
  In1/1 -> Sum/1

== system PC_Simulator_Lib/Comunication_with_visualisation_normal_mode/Subsystem2/Subsystem9 ==
  In1 : Inport
  Constant9 : Constant  Value=Z_init
  Sum : Sum  Inputs=|++
  Out1 : Outport
  wires:
  In1/1 -> Sum/1
  Constant9/1 -> Sum/2
  Sum/1 -> Out1/1

== system PC_Simulator_Lib/Comunication_with_visualisation_normal_mode_new_Version/Maping_Block/Subsystem ==
  Vehicle_1_Vector : Inport
  Vehicle_2_Vector : Inport  Port=2
  Vehicle_3_Vector : Inport  Port=3
  Vehicle_4_Vector : Inport  Port=4
  Vehicle_5_Vector : Inport  Port=5
  Vehicle_6_Vector : Inport  Port=6
  Vehicle_7_Vector : Inport  Port=7
  Vehicle_8_Vector : Inport  Port=8
  Vehicle_9_Vector : Inport  Port=9
  Vehicle_10_Vector : Inport  Port=10
  Vehicle_11_Vector : Inport  Port=11
  Vehicle_12_Vector : Inport  Port=12
  Vehicle_13_Vector : Inport  Port=13
  Vehicle_14_Vector : Inport  Port=14
  Bus Creator : BusCreator  Inputs=14
  Bus Selector : BusSelector  OutputSignals=Vehicle_1_Vector.Vehicle_1_x[m],Vehicle_2_Vector.Vehicle_2_x[m],Vehicle_3_Vector.Vehicle_3_x[m],Vehicle_4_Vector3.Vehicle_4_x[m],Vehicle_5_Vector.Vehicle_5_x[m],Vehicle_6_Vector.Vehicle_6_x[m],Vehicle_7_Vector.Vehicle_7_x[m],Vehicle_8_Vector.Vehicle_8_x[m],Vehicle_9_Vector.Vehicle_9_x[m],Vehicle_10_Vector.Vehicle_10_x[m],Vehicle_11_Vector.Vehicle_11_x[m],Vehicle_12_Vector.Vehicle_12_x[m],Vehicle_13_Vector.Vehicle_13_x[m],Vehicle_14_Vector.Vehicle_14_x[m]
  Bus Selector1 : BusSelector  OutputSignals=Vehicle_1_Vector.Vehicle_1_y[m],Vehicle_2_Vector.Vehicle_2_y[m],Vehicle_3_Vector.Vehicle_3_y[m],Vehicle_4_Vector3.Vehicle_4_y[m],Vehicle_5_Vector.Vehicle_5_y[m],Vehicle_6_Vector.Vehicle_6_y[m],Vehicle_7_Vector.Vehicle_7_y[m],Vehicle_8_Vector.Vehicle_8_y[m],Vehicle_9_Vector.Vehicle_9_y[m],Vehicle_10_Vector.Vehicle_10_y[m],Vehicle_11_Vector.Vehicle_11_y[m],Vehicle_12_Vector.Vehicle_12_y[m],Vehicle_13_Vector.Vehicle_13_y[m],Vehicle_14_Vector.Vehicle_14_y[m]
  Bus Selector2 : BusSelector  OutputSignals=Vehicle_1_Vector.Vehicle_1_z[m],Vehicle_2_Vector.Vehicle_2_z[m],Vehicle_3_Vector.Vehicle_3_z[m],Vehicle_4_Vector3.Vehicle_4_z[m],Vehicle_5_Vector.Vehicle_5_z[m],Vehicle_6_Vector.Vehicle_6_z[m],Vehicle_7_Vector.Vehicle_7_z[m],Vehicle_8_Vector.Vehicle_8_z[m],Vehicle_9_Vector.Vehicle_9_z[m],Vehicle_10_Vector.Vehicle_10_z[m],Vehicle_11_Vector.Vehicle_11_z[m],Vehicle_12_Vector.Vehicle_12_z[m],Vehicle_13_Vector.Vehicle_13_z[m],Vehicle_14_Vector.Vehicle_14_z[m]
  Bus Selector3 : BusSelector  OutputSignals=Vehicle_1_Vector.Vehicle_1_Gear_Angle[deg],Vehicle_2_Vector.Vehicle_2_Gear_Angle[deg],Vehicle_3_Vector.Vehicle_3_Gear_Angle[deg],Vehicle_4_Vector3.Vehicle_4_Gear_Angle[deg],Vehicle_5_Vector.Vehicle_5_Gear_Angle[deg],Vehicle_6_Vector.Vehicle_6_Gear_Angle[deg],Vehicle_7_Vector.Vehicle_7_Gear_Angle[deg],Vehicle_8_Vector.Vehicle_8_Gear_Angle[deg],Vehicle_9_Vector.Vehicle_9_Gear_Angle[deg],Vehicle_10_Vector.Vehicle_10_Gear_Angle[deg],Vehicle_11_Vector.Vehicle_11_Gear_Angle[deg],Vehicle_12_Vector.Vehicle_12_Gear_Angle[deg],Vehicle_13_Vector.Vehicle_13_Gear_Angle[deg],Vehicle_14_Vector.Vehicle_14_Gear_Angle[deg]
  Bus Selector4 : BusSelector  OutputSignals=Vehicle_1_Vector.Vehicle_1_Wheels_Rotation_Angle[deg],Vehicle_2_Vector.Vehicle_2_Wheels_Rotation_Angle[deg],Vehicle_3_Vector.Vehicle_3_Wheels_Rotation_Angle[deg],Vehicle_4_Vector3.Vehicle_4_Wheels_Rotation_Angle[deg],Vehicle_5_Vector.Vehicle_5_Wheels_Rotation_Angle[deg],Vehicle_6_Vector.Vehicle_6_Wheels_Rotation_Angle[deg],Vehicle_7_Vector.Vehicle_7_Wheels_Rotation_Angle[deg],Vehicle_8_Vector.Vehicle_8_Wheels_Rotation_Angle[deg],Vehicle_9_Vector.Vehicle_9_Wheels_Rotation_Angle[deg],Vehicle_10_Vector.Vehicle_10_Wheels_Rotation_Angle[deg],Vehicle_11_Vector.Vehicle_11_Wheels_Rotation_Angle[deg],Vehicle_12_Vector.Vehicle_12_Wheels_Rotation_Angle[deg],Vehicle_13_Vector.Vehicle_13_Wheels_Rotation_Angle[deg],Vehicle_14_Vector.Vehicle_14_Wheels_Rotation_Angle[deg]
  Mux{,1..4} (5 alike) : Mux  Inputs=14
  Fellow_Vehicles_x_Vector_14[m] : Outport
  Fellow_Vehicles_y_Vector_14[m] : Outport  Port=2
  Fellow_Vehicles_z_Vector_14[m] : Outport  Port=3
  Fellow_Vehicles_Gear_Angle_Vector_14[deg] : Outport  Port=4
  Fellow_Vehicles_Wheel_Angle_Vector_14[deg] : Outport  Port=5
  wires:
  Mux4/1 -> Fellow_Vehicles_Wheel_Angle_Vector_14[deg]/1
  Mux3/1 -> Fellow_Vehicles_Gear_Angle_Vector_14[deg]/1
  Mux2/1 -> Fellow_Vehicles_z_Vector_14[m]/1
  Mux1/1 -> Fellow_Vehicles_y_Vector_14[m]/1
  Mux/1 -> Fellow_Vehicles_x_Vector_14[m]/1
  Bus Selector4/1 -> Mux4/1  "<Vehicle_1_Wheels_Rotation_Angle[deg]>"
  Bus Selector4/2 -> Mux4/2  "<Vehicle_2_Wheels_Rotation_Angle[deg]>"
  Bus Selector4/14 -> Mux4/14  "<Vehicle_14_Wheels_Rotation_Angle[deg]>"
  Bus Selector4/3 -> Mux4/3  "<Vehicle_3_Wheels_Rotation_Angle[deg]>"
  Bus Selector4/13 -> Mux4/13  "<Vehicle_13_Wheels_Rotation_Angle[deg]>"
  Bus Selector4/4 -> Mux4/4  "<Vehicle_4_Wheels_Rotation_Angle[deg]>"
  Bus Selector4/12 -> Mux4/12  "<Vehicle_12_Wheels_Rotation_Angle[deg]>"
  Bus Selector4/5 -> Mux4/5  "<Vehicle_5_Wheels_Rotation_Angle[deg]>"
  Bus Selector4/11 -> Mux4/11  "<Vehicle_11_Wheels_Rotation_Angle[deg]>"
  Bus Selector4/6 -> Mux4/6  "<Vehicle_6_Wheels_Rotation_Angle[deg]>"
  Bus Selector4/10 -> Mux4/10  "<Vehicle_10_Wheels_Rotation_Angle[deg]>"
  Bus Selector4/7 -> Mux4/7  "<Vehicle_7_Wheels_Rotation_Angle[deg]>"
  Bus Selector4/9 -> Mux4/9  "<Vehicle_9_Wheels_Rotation_Angle[deg]>"
  Bus Selector4/8 -> Mux4/8  "<Vehicle_8_Wheels_Rotation_Angle[deg]>"
  Bus Creator/1 -> Bus Selector/1, Bus Selector1/1, Bus Selector2/1, Bus Selector3/1, Bus Selector4/1
  Bus Selector3/1 -> Mux3/1  "<Vehicle_1_Gear_Angle[deg]>"
  Bus Selector3/2 -> Mux3/2  "<Vehicle_2_Gear_Angle[deg]>"
  Bus Selector3/14 -> Mux3/14  "<Vehicle_14_Gear_Angle[deg]>"
  Bus Selector3/3 -> Mux3/3  "<Vehicle_3_Gear_Angle[deg]>"
  Bus Selector3/13 -> Mux3/13  "<Vehicle_13_Gear_Angle[deg]>"
  Bus Selector3/4 -> Mux3/4  "<Vehicle_4_Gear_Angle[deg]>"
  Bus Selector3/12 -> Mux3/12  "<Vehicle_12_Gear_Angle[deg]>"
  Bus Selector3/5 -> Mux3/5  "<Vehicle_5_Gear_Angle[deg]>"
  Bus Selector3/11 -> Mux3/11  "<Vehicle_11_Gear_Angle[deg]>"
  Bus Selector3/6 -> Mux3/6  "<Vehicle_6_Gear_Angle[deg]>"
  Bus Selector3/10 -> Mux3/10  "<Vehicle_10_Gear_Angle[deg]>"
  Bus Selector3/7 -> Mux3/7  "<Vehicle_7_Gear_Angle[deg]>"
  Bus Selector3/9 -> Mux3/9  "<Vehicle_9_Gear_Angle[deg]>"
  Bus Selector3/8 -> Mux3/8  "<Vehicle_8_Gear_Angle[deg]>"
  Bus Selector2/1 -> Mux2/1  "<Vehicle_1_z[m]>"
  Bus Selector2/2 -> Mux2/2  "<Vehicle_2_z[m]>"
  Bus Selector2/14 -> Mux2/14  "<Vehicle_14_z[m]>"
  Bus Selector2/3 -> Mux2/3  "<Vehicle_3_z[m]>"
  Bus Selector2/13 -> Mux2/13  "<Vehicle_13_z[m]>"
  Bus Selector2/4 -> Mux2/4  "<Vehicle_4_z[m]>"
  Bus Selector2/12 -> Mux2/12  "<Vehicle_12_z[m]>"
  Bus Selector2/5 -> Mux2/5  "<Vehicle_5_z[m]>"
  Bus Selector2/11 -> Mux2/11  "<Vehicle_11_z[m]>"
  Bus Selector2/6 -> Mux2/6  "<Vehicle_6_z[m]>"
  Bus Selector2/10 -> Mux2/10  "<Vehicle_10_z[m]>"
  Bus Selector2/7 -> Mux2/7  "<Vehicle_7_z[m]>"
  Bus Selector2/9 -> Mux2/9  "<Vehicle_9_z[m]>"
  Bus Selector2/8 -> Mux2/8  "<Vehicle_8_z[m]>"
  Bus Selector1/1 -> Mux1/1  "<Vehicle_1_y[m]>"
  Bus Selector1/2 -> Mux1/2  "<Vehicle_2_y[m]>"
  Bus Selector1/14 -> Mux1/14  "<Vehicle_14_y[m]>"
  Bus Selector1/3 -> Mux1/3  "<Vehicle_3_y[m]>"
  Bus Selector1/13 -> Mux1/13  "<Vehicle_13_y[m]>"
  Bus Selector1/4 -> Mux1/4  "<Vehicle_4_y[m]>"
  Bus Selector1/12 -> Mux1/12  "<Vehicle_12_y[m]>"
  Bus Selector1/5 -> Mux1/5  "<Vehicle_5_y[m]>"
  Bus Selector1/11 -> Mux1/11  "<Vehicle_11_y[m]>"
  Bus Selector1/6 -> Mux1/6  "<Vehicle_6_y[m]>"
  Bus Selector1/10 -> Mux1/10  "<Vehicle_10_y[m]>"
  Bus Selector1/7 -> Mux1/7  "<Vehicle_7_y[m]>"
  Bus Selector1/9 -> Mux1/9  "<Vehicle_9_y[m]>"
  Bus Selector1/8 -> Mux1/8  "<Vehicle_8_y[m]>"
  Bus Selector/1 -> Mux/1  "<Vehicle_1_x[m]>"
  Bus Selector/2 -> Mux/2  "<Vehicle_2_x[m]>"
  Bus Selector/14 -> Mux/14  "<Vehicle_14_x[m]>"
  Bus Selector/3 -> Mux/3  "<Vehicle_3_x[m]>"
  Bus Selector/13 -> Mux/13  "<Vehicle_13_x[m]>"
  Bus Selector/4 -> Mux/4  "<Vehicle_4_x[m]>"
  Bus Selector/12 -> Mux/12  "<Vehicle_12_x[m]>"
  Bus Selector/5 -> Mux/5  "<Vehicle_5_x[m]>"
  Bus Selector/11 -> Mux/11  "<Vehicle_11_x[m]>"
  Bus Selector/6 -> Mux/6  "<Vehicle_6_x[m]>"
  Bus Selector/10 -> Mux/10  "<Vehicle_10_x[m]>"
  Bus Selector/7 -> Mux/7  "<Vehicle_7_x[m]>"
  Bus Selector/9 -> Mux/9  "<Vehicle_9_x[m]>"
  Bus Selector/8 -> Mux/8  "<Vehicle_8_x[m]>"
  Vehicle_14_Vector/1 -> Bus Creator/14
  Vehicle_12_Vector/1 -> Bus Creator/12
  Vehicle_11_Vector/1 -> Bus Creator/11
  Vehicle_9_Vector/1 -> Bus Creator/9
  Vehicle_10_Vector/1 -> Bus Creator/10
  Vehicle_13_Vector/1 -> Bus Creator/13
  Vehicle_8_Vector/1 -> Bus Creator/8
  Vehicle_7_Vector/1 -> Bus Creator/7
  Vehicle_6_Vector/1 -> Bus Creator/6
  Vehicle_5_Vector/1 -> Bus Creator/5
  Vehicle_4_Vector/1 -> Bus Creator/4
  Vehicle_3_Vector/1 -> Bus Creator/3
  Vehicle_2_Vector/1 -> Bus Creator/2
  Vehicle_1_Vector/1 -> Bus Creator/1

== system PC_Simulator_Lib/Comunication_with_visualisation_normal_mode_new_Version/Subsystem2/Subsystem ==
  In1 : Inport
  Constant9 : Constant  Value=0.8
  Sum : Sum  Inputs=|++
  Out1 : Outport
  wires:
  Sum/1 -> Out1/1
  Constant9/1 -> Sum/2
  In1/1 -> Sum/1

== system PC_Simulator_Lib/Comunication_with_visualisation_normal_mode_new_Version/Subsystem2/Subsystem1 ==
  In1 : Inport
  Constant9 : Constant  Value=Z_init
  Sum : Sum  Inputs=|++
  Out1 : Outport
  wires:
  In1/1 -> Sum/1
  Constant9/1 -> Sum/2
  Sum/1 -> Out1/1

== system PC_Simulator_Lib/Comunication_with_visualisation_normal_mode_new_Version/Subsystem2/Subsystem10 ==
  In1 : Inport
  Constant9 : Constant  Value=Z_init
  Sum : Sum  Inputs=|++
  Out1 : Outport
  wires:
  In1/1 -> Sum/1
  Constant9/1 -> Sum/2
  Sum/1 -> Out1/1

== system PC_Simulator_Lib/Comunication_with_visualisation_normal_mode_new_Version/Subsystem2/Subsystem11 ==
  v[m|s] : Inport
  Gain : Gain  Gain=1/radiusWheel
  Integrator : Integrator
  Wheels_Rotation_Angle[rad] : Outport
  wires:
  Gain/1 -> Integrator/1
  v[m|s]/1 -> Gain/1
  Integrator/1 -> Wheels_Rotation_Angle[rad]/1

== system PC_Simulator_Lib/Comunication_with_visualisation_normal_mode_new_Version/Subsystem2/Subsystem12 ==
  v[m|s] : Inport
  Gain : Gain  Gain=1/radiusWheel
  Integrator : Integrator
  Wheels_Rotation_Angle[rad] : Outport
  wires:
  Integrator/1 -> Wheels_Rotation_Angle[rad]/1
  v[m|s]/1 -> Gain/1
  Gain/1 -> Integrator/1

== system PC_Simulator_Lib/Comunication_with_visualisation_normal_mode_new_Version/Subsystem2/Subsystem13 ==
  v[m|s] : Inport
  Gain : Gain  Gain=1/radiusWheel
  Integrator : Integrator
  Wheels_Rotation_Angle[rad] : Outport
  wires:
  Gain/1 -> Integrator/1
  v[m|s]/1 -> Gain/1
  Integrator/1 -> Wheels_Rotation_Angle[rad]/1

== system PC_Simulator_Lib/Comunication_with_visualisation_normal_mode_new_Version/Subsystem2/Subsystem14 ==
  v[m|s] : Inport
  Gain : Gain  Gain=1/radiusWheel
  Integrator : Integrator
  Wheels_Rotation_Angle[rad] : Outport
  wires:
  Integrator/1 -> Wheels_Rotation_Angle[rad]/1
  v[m|s]/1 -> Gain/1
  Gain/1 -> Integrator/1

== system PC_Simulator_Lib/Comunication_with_visualisation_normal_mode_new_Version/Subsystem2/Subsystem15 ==
  v[m|s] : Inport
  Gain : Gain  Gain=1/radiusWheel
  Integrator : Integrator
  Wheels_Rotation_Angle[rad] : Outport
  wires:
  Gain/1 -> Integrator/1
  v[m|s]/1 -> Gain/1
  Integrator/1 -> Wheels_Rotation_Angle[rad]/1

== system PC_Simulator_Lib/Comunication_with_visualisation_normal_mode_new_Version/Subsystem2/Subsystem16 ==
  v[m|s] : Inport
  Gain : Gain  Gain=1/radiusWheel
  Integrator : Integrator
  Wheels_Rotation_Angle[rad] : Outport
  wires:
  Integrator/1 -> Wheels_Rotation_Angle[rad]/1
  v[m|s]/1 -> Gain/1
  Gain/1 -> Integrator/1

== system PC_Simulator_Lib/Comunication_with_visualisation_normal_mode_new_Version/Subsystem2/Subsystem17 ==
  v[m|s] : Inport
  Gain : Gain  Gain=1/radiusWheel
  Integrator : Integrator
  Wheels_Rotation_Angle[rad] : Outport
  wires:
  Gain/1 -> Integrator/1
  v[m|s]/1 -> Gain/1
  Integrator/1 -> Wheels_Rotation_Angle[rad]/1

== system PC_Simulator_Lib/Comunication_with_visualisation_normal_mode_new_Version/Subsystem2/Subsystem18 ==
  v[m|s] : Inport
  Gain : Gain  Gain=1/radiusWheel
  Integrator : Integrator
  Wheels_Rotation_Angle[rad] : Outport
  wires:
  Integrator/1 -> Wheels_Rotation_Angle[rad]/1
  v[m|s]/1 -> Gain/1
  Gain/1 -> Integrator/1

== system PC_Simulator_Lib/Comunication_with_visualisation_normal_mode_new_Version/Subsystem2/Subsystem19 ==
  v[m|s] : Inport
  Gain : Gain  Gain=1/radiusWheel
  Integrator : Integrator
  Wheels_Rotation_Angle[rad] : Outport
  wires:
  Gain/1 -> Integrator/1
  v[m|s]/1 -> Gain/1
  Integrator/1 -> Wheels_Rotation_Angle[rad]/1

== system PC_Simulator_Lib/Comunication_with_visualisation_normal_mode_new_Version/Subsystem2/Subsystem2 ==
  In1 : Inport
  Constant9 : Constant  Value=Z_init
  Sum : Sum  Inputs=|++
  Out1 : Outport
  wires:
  Sum/1 -> Out1/1
  Constant9/1 -> Sum/2
  In1/1 -> Sum/1

== system PC_Simulator_Lib/Comunication_with_visualisation_normal_mode_new_Version/Subsystem2/Subsystem20 ==
  v[m|s] : Inport
  Gain : Gain  Gain=1/radiusWheel
  Integrator : Integrator
  Wheels_Rotation_Angle[rad] : Outport
  wires:
  Integrator/1 -> Wheels_Rotation_Angle[rad]/1
  v[m|s]/1 -> Gain/1
  Gain/1 -> Integrator/1

== system PC_Simulator_Lib/Comunication_with_visualisation_normal_mode_new_Version/Subsystem2/Subsystem4 ==
  In1 : Inport
  Constant9 : Constant  Value=Z_init
  Sum : Sum  Inputs=|++
  Out1 : Outport
  wires:
  In1/1 -> Sum/1
  Constant9/1 -> Sum/2
  Sum/1 -> Out1/1

== system PC_Simulator_Lib/Comunication_with_visualisation_normal_mode_new_Version/Subsystem2/Subsystem5 ==
  In1 : Inport
  Constant9 : Constant  Value=Z_init
  Sum : Sum  Inputs=|++
  Out1 : Outport
  wires:
  Sum/1 -> Out1/1
  Constant9/1 -> Sum/2
  In1/1 -> Sum/1

== system PC_Simulator_Lib/Comunication_with_visualisation_normal_mode_new_Version/Subsystem2/Subsystem6 ==
  In1 : Inport
  Constant9 : Constant  Value=Z_init
  Sum : Sum  Inputs=|++
  Out1 : Outport
  wires:
  In1/1 -> Sum/1
  Constant9/1 -> Sum/2
  Sum/1 -> Out1/1
